simulink model "Data"  (R2023b)
settings: Solver=VariableStepAuto  StartTime=0.0  StopTime=10.0  RelTol=1e-3
settings Model: Creator=visha  LastModifiedBy=visha
settings OptimizationCC: DefaultParameterBehavior=Inlined

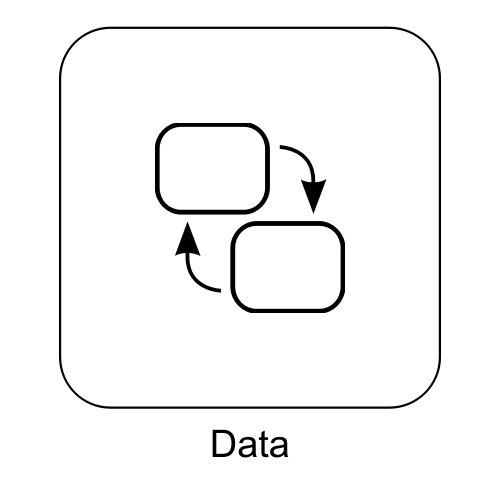
[thumbnail: Simulink's stored preview of the top-level diagram]
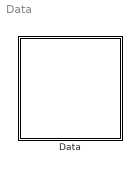
== system Data ==
  Data : Stateflow chart  TreatAsAtomicUnit=on

== stateflow chart Data/Data ==
  state Data
  state StandBy
  state RESET
  (default) -> Data
  StandBy -> RESET
  Data -> StandBy
